simulink model "language"  (Simulink 7.6)
settings: Solver=FixedStepDiscrete  StartTime=0.0  StopTime=10.0  FixedStep=1  RelTol=1e-3
settings Model: Creator=ksmyth  LastModifiedBy=c2wt
settings OptimizationCC: InitFltsAndDblsToZero=on
settings DebuggingCC: SaveWithParameterizedLinksMsg=none  StrictBusMsg=Warning
settings SFSimCC: SimParseCustomCode=off
settings GRTTargetCC: TargetFcnLib=ansi_tfl_tmw.mat

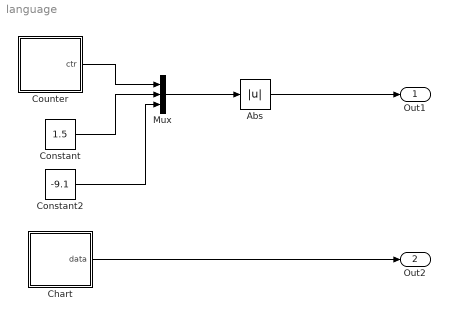
== system language ==
  Abs : Abs
  Chart : Stateflow chart  TreatAsAtomicUnit=on
  Constant : Constant  Value=1.5
  Constant2 : Constant  Value=-9.1
  Counter : Stateflow chart  TreatAsAtomicUnit=on
  Mux : Mux  Inputs=3
  Out1 : Outport
  Out2 : Outport  Port=2
  wires:
  Counter/1(ctr) -> Mux/1
  Mux/1 -> Abs/1
  Abs/1 -> Out1/1
  Constant/1 -> Mux/2
  Chart/1(data) -> Out2/1
  Constant2/1 -> Mux/3

== stateflow chart Counter ==
  state s1
  (default) -> s1
  s1 -> s1 [order 1] : /* increment counter */
      | [ctr < 4]
      | {
      |   /* test comment */ctr++;/* second test comment */
      | }
  s1 -> s1 [order 2] : [ctr >= 4] /
      | % reset counter
      | ctr -= 6;
  data: ctr output double =1

== stateflow chart Chart ==
  state State1
  State1 -> State1 [order 1] : [ data[ 0 ][ 0 ] > 0 ] / data[ 0 ][ 0 ] = 0;data[ 0 ][ 1 ] += 2
  State1 -> State1 [order 2] : [ data[ 0 ][ 1 ] > 0 ] // SHOULD BE WITH CONDITION-ACTION
      | / data[ 0 ][ 1 ] = 0;data[ 1 ][ 0 ] += 3
  State1 -> State1 [order 3] : [ data[ 1 ][ 0 ] > 0 ] / data[ 1 ][ 0 ] = 0;data[ 1 ][ 1 ] += 4
  State1 -> State1 [order 4] : / data[ 0 ][ 0 ]++
  (default) -> State1
  data: data output double size=[ 2 2 ] =[ 0 0 ; 0 0 ]
